simulink model "Encryption"  (R2020b)
settings: Solver=VariableStepAuto  StartTime=0.0  StopTime=10.0  RelTol=1e-3
settings Model: Creator=macra  LastModifiedBy=macra

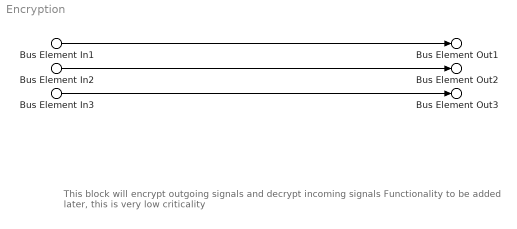
== system Encryption ==
  note: This block will encrypt outgoing signals and decrypt incoming signals
      |
      | Functionality to be added later, this is very low criticality
  Bus Element In1 : Inport  PortName=Flight Command
  Bus Element In2 : Inport  Port=2  PortName=Encrypted Data From Drone
  Bus Element In3 : Inport  Port=3  PortName=Encrypted Video From Drone
  Bus Element Out2 : Outport  PortName=Decrypted Data From Drone
  Bus Element Out3 : Outport  Port=2  PortName=Decrypted Video From Drone
  Bus Element Out1 : Outport  Port=3  PortName=Encrypted Data To Drone
  wires:
  Bus Element In1/1 -> Bus Element Out1/1
  Bus Element In2/1 -> Bus Element Out2/1
  Bus Element In3/1 -> Bus Element Out3/1
